simulink model "EKF"  (R2020a)
settings: Solver=VariableStepAuto  StartTime=0.0  StopTime=160  RelTol=1e-3
model workspace (MAT data in the model file):
  Mav0_init = Simulink.Parameter
  Mav0_init.Value = [0.515356; 1.996773; 0.971104; -0.002276; -0.009616; -0.005214; 0.161996; 0.789985; -0.205376; 0.554528; 0; 0; 0; 0; 0; 0; 1; 1; 1; 1; 1; 1; 0; 0; -9.81]
  Mav0_init.DataType = 'auto'
  Mav0_init.Dimensions = [25 1]
  dT = Simulink.Parameter
  dT.Value = 0.01
  dT.DataType = 'auto'
  dT.Dimensions = [1 1]
  g_n = Simulink.Parameter
  g_n.Value = -9.807
  g_n.DataType = 'auto'
  g_n.Dimensions = [1 1]
  sig_a = Simulink.Parameter
  sig_a.Value = 0.4
  sig_a.DataType = 'auto'
  sig_a.Dimensions = [1 1]
  sig_w = Simulink.Parameter
  sig_w.Value = 0.03
  sig_w.DataType = 'auto'
  sig_w.Dimensions = [1 1]
  sigma_l = Simulink.Parameter
  sigma_l.Value = 0.3
  sigma_l.DataType = 'auto'
  sigma_l.Dimensions = [1 1]
  sigma_q = Simulink.Parameter
  sigma_q.Value = 0.05
  sigma_q.DataType = 'auto'
  sigma_q.Dimensions = [1 1]
  sigma_u = Simulink.Parameter
  sigma_u.Value = 0.05
  sigma_u.DataType = 'auto'
  sigma_u.Dimensions = [1 1]
  sigma_u_res = Simulink.Parameter
  sigma_u_res.Value = 0.05
  sigma_u_res.DataType = 'auto'
  sigma_u_res.Dimensions = [1 1]
undefined symbols (not defined in the file or in its folder): Init, no_switchoff
libraries: commchan3 x3
settings Model: OrderedModelArguments=off  Creator=lorenzocollodi  LastModifiedBy=lorenzocollodi

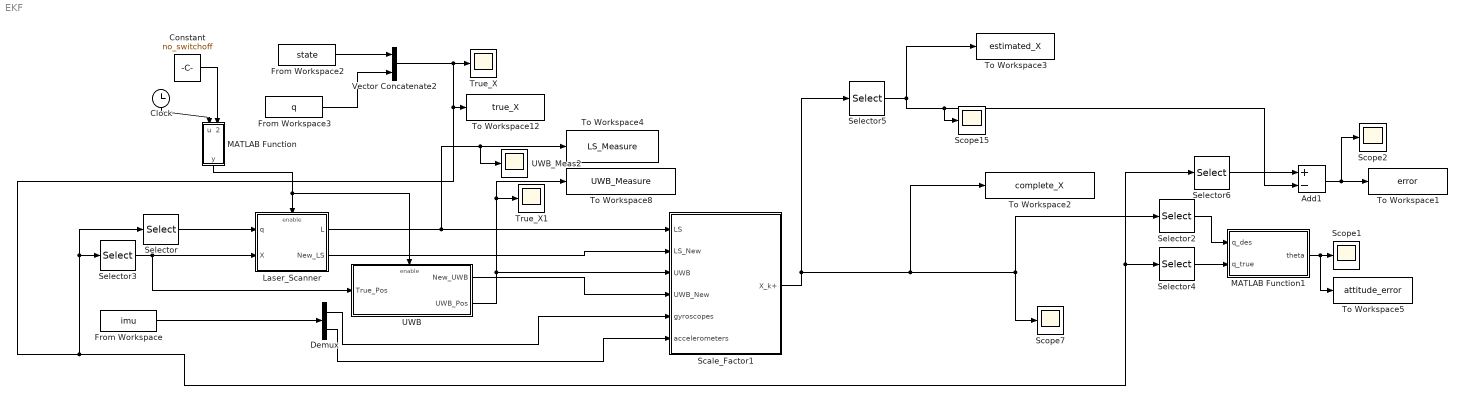
== system EKF ==
  Add1 : Sum  Inputs=+-
  Clock : Clock
  Constant : Constant  Value=no_switchoff
  Demux : Demux  Outputs=2
  From Workspace : FromWorkspace  VariableName=imu
  From Workspace2 : FromWorkspace  VariableName=state
  From Workspace3 : FromWorkspace  VariableName=q  ZeroCross=off
  Laser_Scanner : Subsystem
  MATLAB Function : MATLAB Function  TreatAsAtomicUnit=on
  MATLAB Function1 : MATLAB Function  TreatAsAtomicUnit=on
  Scale_Factor1 : Subsystem
  Scope{1..2,7,15} (4 alike) : Scope
  Selector : Selector  InputPortWidth=10  IndexOptions=Index vector (dialog)  Indices=[7:10]  OutputSizes=1
  Selector2 : Selector  InputPortWidth=25  IndexOptions=Index vector (dialog)  Indices=[7:10]  OutputSizes=1
  Selector3 : Selector  InputPortWidth=10  IndexOptions=Index vector (dialog)  Indices=[1 2 3]  OutputSizes=1
  Selector4 : Selector  InputPortWidth=10  IndexOptions=Index vector (dialog)  Indices=[7:10]  OutputSizes=1
  Selector5 : Selector  InputPortWidth=25  IndexOptions=Index vector (dialog)  Indices=[1:6]  OutputSizes=1
  Selector6 : Selector  InputPortWidth=10  IndexOptions=Index vector (dialog)  Indices=[1:6]  OutputSizes=1
  To Workspace1 : ToWorkspace  VariableName=error  SaveFormat=Timeseries  SampleTime=0.01
  To Workspace12 : ToWorkspace  VariableName=true_X  SaveFormat=Timeseries  SampleTime=0.01
  To Workspace2 : ToWorkspace  VariableName=complete_X  SaveFormat=Timeseries  SampleTime=0.01
  To Workspace3 : ToWorkspace  VariableName=estimated_X  SaveFormat=Timeseries  SampleTime=0.01
  To Workspace4 : ToWorkspace  VariableName=LS_Measure  SaveFormat=Timeseries  SampleTime=0.01
  To Workspace5 : ToWorkspace  VariableName=attitude_error  SaveFormat=Timeseries  SampleTime=0.01
  To Workspace8 : ToWorkspace  VariableName=UWB_Measure  SaveFormat=Timeseries  SampleTime=0.01
  True_X : Scope
  True_X1 : Scope
  UWB : Subsystem
  UWB_Meas2 : Scope
  Vector Concatenate2 : Concatenate
  wires:
  UWB/1(New_UWB) -> Scale_Factor1/4(UWB_New)
  Selector5/1 -> To Workspace3/1, Scope15/1, Add1/2
  Scale_Factor1/1(X_k+) -> To Workspace2/1, Scope7/1, Selector2/1, Selector5/1
  Laser_Scanner/2(New_LS) -> Scale_Factor1/2(LS_New)
  UWB/2(UWB_Pos) -> True_X1/1, To Workspace8/1, Scale_Factor1/3(UWB)
  Add1/1 -> Scope2/1, To Workspace1/1
  From Workspace2/1 -> Vector Concatenate2/1
  Demux/1 -> Scale_Factor1/5(gyroscopes)
  Selector4/1 -> MATLAB Function1/2(q_true)
  Selector6/1 -> Add1/1
  MATLAB Function/1(y) -> UWB/Enable, Laser_Scanner/Enable
  Demux/2 -> Scale_Factor1/6(accelerometers)
  Selector3/1 -> UWB/1(True_Pos), Laser_Scanner/2(X)
  Laser_Scanner/1(L) -> To Workspace4/1, UWB_Meas2/1, Scale_Factor1/1(LS)
  Selector2/1 -> MATLAB Function1/1(q_des)
  Vector Concatenate2/1 -> Selector6/1, Selector4/1, Selector3/1, Selector/1, To Workspace12/1, True_X/1
  MATLAB Function1/1(theta) -> To Workspace5/1, Scope1/1
  From Workspace3/1 -> Vector Concatenate2/2
  From Workspace/1 -> Demux/1
  Clock/1 -> MATLAB Function/1(u)
  Selector/1 -> Laser_Scanner/1(q)
  Constant/1 -> MATLAB Function/2(no_switchoff)

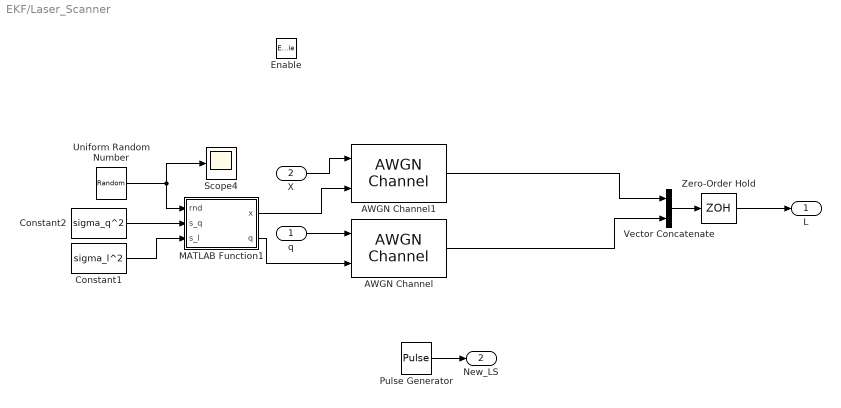
== system EKF/Laser_Scanner ==
  q : Inport  SampleTime=0.005
  X : Inport  Port=2  SampleTime=0.005
  Enable : EnablePort  StatesWhenEnabling=reset
  AWGN Channel : commchan3/AWGN Channel  InputProcessing=Columns as channels (frame based)  seed=53  noiseMode=Variance from port  EbNodB=10  EsNodB=10  SNRdB=10  bitsPerSym=1  Ps=1  Tsym=1  variance=sigma_q^2
  AWGN Channel1 : commchan3/AWGN Channel  InputProcessing=Columns as channels (frame based)  seed=123  noiseMode=Variance from port  EbNodB=10  EsNodB=10  SNRdB=10  bitsPerSym=1  Ps=1  Tsym=1  variance=sigma_l^2
  Constant1 : Constant  Value=sigma_l^2
  Constant2 : Constant  Value=sigma_q^2
  MATLAB Function1 : MATLAB Function  TreatAsAtomicUnit=on
  Pulse Generator : DiscretePulseGenerator  PulseType=Time based  Period=0.1  PulseWidth=5  PhaseDelay=0.1
  Scope4 : Scope
  Uniform Random Number : UniformRandomNumber  Minimum=0  SampleTime=0.1
  Vector Concatenate : Concatenate
  Zero-Order Hold : ZeroOrderHold  SampleTime=0.1
  L : Outport  SampleTime=0.005
  New_LS : Outport  Port=2  SampleTime=0.005  InitialOutput=0
  wires:
  X/1 -> AWGN Channel1/1
  Pulse Generator/1 -> New_LS/1
  Vector Concatenate/1 -> Zero-Order Hold/1
  AWGN Channel1/1 -> Vector Concatenate/1
  Zero-Order Hold/1 -> L/1
  Uniform Random Number/1 -> Scope4/1, MATLAB Function1/1(rnd)
  MATLAB Function1/1(x) -> AWGN Channel1/2
  MATLAB Function1/2(q) -> AWGN Channel/2
  q/1 -> AWGN Channel/1
  AWGN Channel/1 -> Vector Concatenate/2
  Constant2/1 -> MATLAB Function1/2(s_q)
  Constant1/1 -> MATLAB Function1/3(s_l)

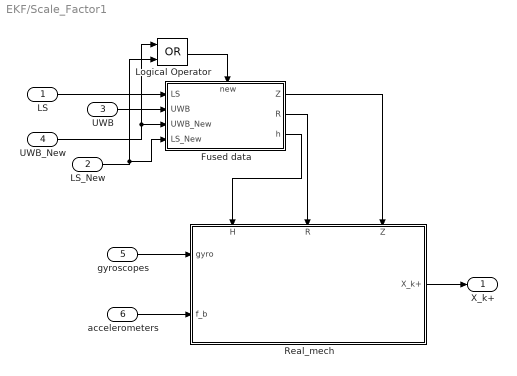
== system EKF/Scale_Factor1 ==
  LS : Inport  SampleTime=0.005
  LS_New : Inport  Port=2  SampleTime=0.005
  UWB : Inport  Port=3  SampleTime=0.005
  UWB_New : Inport  Port=4  SampleTime=0.005
  gyroscopes : Inport  Port=5  SampleTime=0.005
  accelerometers : Inport  Port=6  SampleTime=0.005
  Fused data : Subsystem
      settings: PortSchema="{\"entries\":[{\"content\":{\"sides\":[{\"content\":{\"connectorIds\":[\"In1\",\"In2\",\"In3\",\"In4\"]},\"type\":\"ConnectorPlacement.EquallySpacedRectSide\",\"uuid\":\"3f1f864a-0375-4254-b0e5-a3ccef78d94b\"},{\"content\":{\"connectorIds\":[\"Out1\",\"Out2\",\"Out3\"],\"side\":\"RIGHT\"},\"type\":\"ConnectorPlacement.EquallySpacedRectSide\",\"uuid\":\"a0a53594-1cb6-457a-b6d6-466f13dde723\"},{\"content\":{\"connectorIds\":[\"In5\"],\"side\":\"TOP\"},\"type\":\"ConnectorPlacement.EquallySpacedRectSide\",\"uuid\":\"6845f56e-1f73-40df-9b1b-67b0b5fba5c0\"}]},\"type\":\"ConnectorPlacement.EquallySpacedConnector\",\"uuid\":\"e6a25399-179c-4a75-bf96-00b096d7750c\"}],\"packageUris\":[\"http://schema.mathworks.com/mf0/Connector/19700101\"],\"version\":\"1.0\"}"
  Logical Operator : Logic  Operator=OR  AllPortsSameDT=off  OutDataTypeStr=boolean
  Real_mech : Subsystem
      settings: PortSchema="{\"entries\":[{\"content\":{\"sides\":[{\"content\":{\"connectorIds\":[\"In1\",\"In2\"]},\"type\":\"ConnectorPlacement.EquallySpacedRectSide\",\"uuid\":\"f4a09739-15c6-4b87-9129-8eaded998bc8\"},{\"content\":{\"connectorIds\":[\"Out1\"],\"side\":\"RIGHT\"},\"type\":\"ConnectorPlacement.EquallySpacedRectSide\",\"uuid\":\"b65aee05-6731-4b1e-8841-18a97eaa40b2\"},{\"content\":{\"connectorIds\":[\"In3\",\"In4\",\"In5\"],\"side\":\"TOP\"},\"type\":\"ConnectorPlacement.EquallySpacedRectSide\",\"uuid\":\"6689e3e2-b7bb-4bc5-8dd6-d15d67eac7bb\"}]},\"type\":\"ConnectorPlacement.EquallySpacedConnector\",\"uuid\":\"d04e917e-36a5-4a97-9f44-5590d0d9db30\"}],\"packageUris\":[\"http://schema.mathworks.com/mf0/Connector/19700101\"],\"version\":\"1.0\"}"
  X_k+ : Outport  SampleTime=0.005
  wires:
  UWB/1 -> Fused data/2(UWB)
  accelerometers/1 -> Real_mech/2(f_b)
  Real_mech/1(X_k+) -> X_k+/1
  gyroscopes/1 -> Real_mech/1(gyro)
  LS_New/1 -> Fused data/4(LS_New), Logical Operator/2
  UWB_New/1 -> Logical Operator/1, Fused data/3(UWB_New)
  Fused data/1(Z) -> Real_mech/5(Z)
  Fused data/2(R) -> Real_mech/4(R)
  Fused data/3(h) -> Real_mech/3(H)
  LS/1 -> Fused data/1(LS)
  Logical Operator/1 -> Fused data/5(new)

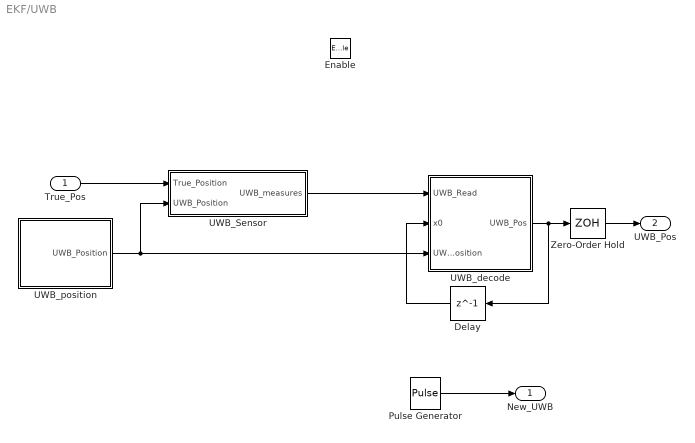
== system EKF/UWB ==
  True_Pos : Inport  SampleTime=0.005
  Enable : EnablePort
  Delay : Delay  DelayLength=1  InitialCondition=[0; 0; 0]  SampleTime=0.1
  Pulse Generator : DiscretePulseGenerator  PulseType=Time based  Period=0.1  PulseWidth=5  PhaseDelay=0.1
  UWB_Sensor : Subsystem
  UWB_decode : Subsystem
  UWB_position : Subsystem
  Zero-Order Hold : ZeroOrderHold  SampleTime=0.1
  New_UWB : Outport  SampleTime=0.005  InitialOutput=0
  UWB_Pos : Outport  Port=2  SampleTime=0.005
  wires:
  True_Pos/1 -> UWB_Sensor/1(True_Position)
  UWB_Sensor/1(UWB_measures) -> UWB_decode/1(UWB_Read)
  UWB_position/1(UWB_Position) -> UWB_Sensor/2(UWB_Position), UWB_decode/3(UWB_Position)
  Delay/1 -> UWB_decode/2(x0)
  UWB_decode/1(UWB_Pos) -> Zero-Order Hold/1, Delay/1
  Pulse Generator/1 -> New_UWB/1
  Zero-Order Hold/1 -> UWB_Pos/1

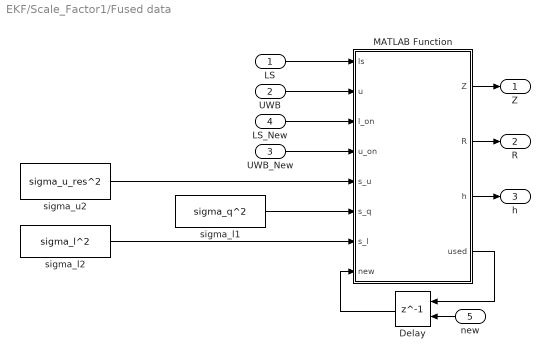
== system EKF/Scale_Factor1/Fused data ==
  LS : Inport  SampleTime=0.005
  UWB : Inport  Port=2  SampleTime=0.005
  UWB_New : Inport  Port=3  SampleTime=0.005
  LS_New : Inport  Port=4  SampleTime=0.005
  new : Inport  Port=5  SampleTime=0.005
  Delay : Delay  DelayLength=1  InitialCondition=1  ExternalReset=Rising  SampleTime=0.005
      settings: InputPortMap=u0,r5
  MATLAB Function : MATLAB Function  TreatAsAtomicUnit=on
  sigma_l1 : Constant  Value=sigma_q^2
  sigma_l2 : Constant  Value=sigma_l^2
  sigma_u2 : Constant  Value=sigma_u_res^2
  Z : Outport  SampleTime=0.005
  R : Outport  Port=2  SampleTime=0.005
  h : Outport  Port=3  SampleTime=0.005
  wires:
  LS/1 -> MATLAB Function/1(ls)
  UWB/1 -> MATLAB Function/2(u)
  UWB_New/1 -> MATLAB Function/4(u_on)
  sigma_u2/1 -> MATLAB Function/5(s_u)
  sigma_l2/1 -> MATLAB Function/7(s_l)
  MATLAB Function/1(Z) -> Z/1
  MATLAB Function/2(R) -> R/1
  MATLAB Function/3(h) -> h/1
  MATLAB Function/4(used) -> Delay/1
  Delay/1 -> MATLAB Function/8(new)
  new/1 -> Delay/2
  sigma_l1/1 -> MATLAB Function/6(s_q)
  LS_New/1 -> MATLAB Function/3(l_on)

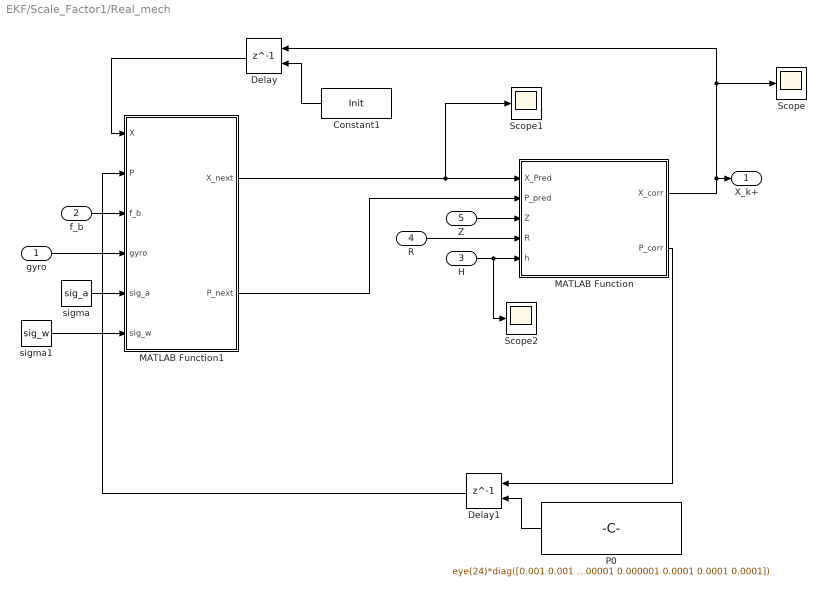
== system EKF/Scale_Factor1/Real_mech ==
  gyro : Inport  SampleTime=0.005
  f_b : Inport  Port=2  SampleTime=0.005
  H : Inport  Port=3  PortDimensions=[7, 25]  SampleTime=0.005
  R : Inport  Port=4  PortDimensions=[7,7]  SampleTime=0.005
  Z : Inport  Port=5  SampleTime=0.005
  Constant1 : Constant  Value=Init
  Delay : Delay  DelayLength=1  InitialConditionSource=Input port  InitialCondition=[0.515356;1.996773;0.971104;-0.002276;-0.009616;-0.005214; 0; 0; -9.81]  SampleTime=0.005
      settings: InputPortMap=u0,p4
  Delay1 : Delay  DelayLength=1  InitialConditionSource=Input port  InitialCondition=0  SampleTime=0.005
      settings: InputPortMap=u0,p4
  MATLAB Function : MATLAB Function  TreatAsAtomicUnit=on
  MATLAB Function1 : MATLAB Function  TreatAsAtomicUnit=on
  P0 : Constant  Value=eye(24)*diag([0.001 0.001 0.001 0.001 0.001 0.001 0.0001 0.0001 0.0001 0.0001 0.001 0.001 0.001 0.000001 0.000001 0.0000001 0.000001 0.000001 0.000001 0.000001 0.000001 0.0001 0.0001 0.0001])
  Scope : Scope
  Scope1 : Scope
  Scope2 : Scope
  sigma : Constant  Value=sig_a  SampleTime=0.01
  sigma1 : Constant  Value=sig_w  SampleTime=0.01
  X_k+ : Outport  SampleTime=0.005
  wires:
  sigma1/1 -> MATLAB Function1/6(sig_w)
  MATLAB Function/1(X_corr) -> Delay/1, Scope/1, X_k+/1
  Delay/1 -> MATLAB Function1/1(X)
  Delay1/1 -> MATLAB Function1/2(P)
  gyro/1 -> MATLAB Function1/4(gyro)
  P0/1 -> Delay1/2
  R/1 -> MATLAB Function/4(R)
  Z/1 -> MATLAB Function/3(Z)
  H/1 -> Scope2/1, MATLAB Function/5(h)
  Constant1/1 -> Delay/2
  f_b/1 -> MATLAB Function1/3(f_b)
  MATLAB Function1/2(P_next) -> MATLAB Function/2(P_pred)
  sigma/1 -> MATLAB Function1/5(sig_a)
  MATLAB Function1/1(X_next) -> Scope1/1, MATLAB Function/1(X_Pred)
  MATLAB Function/2(P_corr) -> Delay1/1

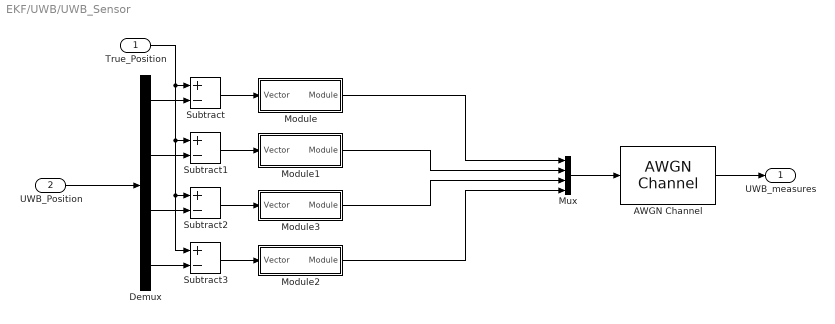
== system EKF/UWB/UWB_Sensor ==
  True_Position : Inport
  UWB_Position : Inport  Port=2
  AWGN Channel : commchan3/AWGN Channel  InputProcessing=Columns as channels (frame based)  seed=13561  noiseMode=Variance from mask  EbNodB=10  EsNodB=10  SNRdB=10  bitsPerSym=1  Ps=1  Tsym=1  variance=sigma_u^2
  Demux : Demux
  Module : Subsystem
  Module1 : Subsystem
  Module2 : Subsystem
  Module3 : Subsystem
  Mux : Mux
  Subtract{,1..3} (4 alike) : Sum  Inputs=+-
  UWB_measures : Outport  PortDimensions=4
  wires:
  UWB_Position/1 -> Demux/1
  Demux/1 -> Subtract/2
  Demux/4 -> Subtract3/2
  Demux/3 -> Subtract2/2
  Demux/2 -> Subtract1/2
  True_Position/1 -> Subtract2/1, Subtract3/1, Subtract1/1, Subtract/1
  Subtract/1 -> Module/1(Vector)
  Subtract3/1 -> Module2/1(Vector)
  Subtract2/1 -> Module3/1(Vector)
  Subtract1/1 -> Module1/1(Vector)
  Mux/1 -> AWGN Channel/1
  AWGN Channel/1 -> UWB_measures/1
  Module/1(Module) -> Mux/1
  Module1/1(Module) -> Mux/2
  Module3/1(Module) -> Mux/3
  Module2/1(Module) -> Mux/4

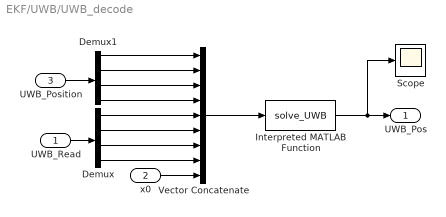
== system EKF/UWB/UWB_decode ==
  UWB_Read : Inport  PortDimensions=4  SampleTime=10*dT
  x0 : Inport  Port=2  PortDimensions=3  SampleTime=10*dT
  UWB_Position : Inport  Port=3  SampleTime=10*dT
  Demux : Demux
  Demux1 : Demux
  Interpreted MATLAB Function : MATLABFcn  MATLABFcn=solve_UWB  OutputDimensions=3
  Scope : Scope
  Vector Concatenate : Concatenate  NumInputs=9
  UWB_Pos : Outport  PortDimensions=3  SampleTime=0.1
  wires:
  UWB_Read/1 -> Demux/1
  Demux1/1 -> Vector Concatenate/1
  Demux1/2 -> Vector Concatenate/2
  Demux1/3 -> Vector Concatenate/3
  Demux1/4 -> Vector Concatenate/4
  Demux/1 -> Vector Concatenate/5
  Demux/2 -> Vector Concatenate/6
  Demux/3 -> Vector Concatenate/7
  Demux/4 -> Vector Concatenate/8
  Interpreted MATLAB Function/1 -> Scope/1, UWB_Pos/1
  x0/1 -> Vector Concatenate/9
  UWB_Position/1 -> Demux1/1
  Vector Concatenate/1 -> Interpreted MATLAB Function/1

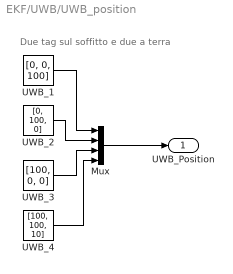
== system EKF/UWB/UWB_position ==
  note: Due tag sul soffitto e due a terra
  Mux : Mux
  UWB_1 : Constant  Value=[0, 0, 100]
  UWB_2 : Constant  Value=[0, 100, 0]
  UWB_3 : Constant  Value=[100, 0, 0]
  UWB_4 : Constant  Value=[100, 100, 10]
  UWB_Position : Outport
  wires:
  UWB_3/1 -> Mux/3
  Mux/1 -> UWB_Position/1
  UWB_4/1 -> Mux/4
  UWB_1/1 -> Mux/1
  UWB_2/1 -> Mux/2

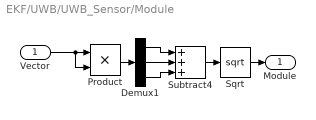
== system EKF/UWB/UWB_Sensor/Module ==
  Vector : Inport
  Demux1 : Demux  Outputs=3
  Product : Product
  Sqrt : Sqrt  SaturateOnIntegerOverflow=on
  Subtract4 : Sum  Inputs=+++
  Module : Outport  PortDimensions=1
  wires:
  Subtract4/1 -> Sqrt/1
  Vector/1 -> Product/2, Product/1
  Product/1 -> Demux1/1
  Demux1/1 -> Subtract4/1
  Demux1/3 -> Subtract4/3
  Demux1/2 -> Subtract4/2
  Sqrt/1 -> Module/1

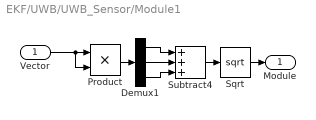
== system EKF/UWB/UWB_Sensor/Module1 ==
  Vector : Inport
  Demux1 : Demux  Outputs=3
  Product : Product
  Sqrt : Sqrt  SaturateOnIntegerOverflow=on
  Subtract4 : Sum  Inputs=+++
  Module : Outport  PortDimensions=1
  wires:
  Demux1/3 -> Subtract4/3
  Subtract4/1 -> Sqrt/1
  Product/1 -> Demux1/1
  Sqrt/1 -> Module/1
  Demux1/1 -> Subtract4/1
  Vector/1 -> Product/2, Product/1
  Demux1/2 -> Subtract4/2

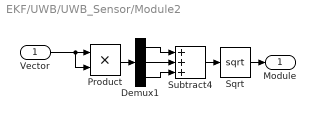
== system EKF/UWB/UWB_Sensor/Module2 ==
  Vector : Inport
  Demux1 : Demux  Outputs=3
  Product : Product
  Sqrt : Sqrt  SaturateOnIntegerOverflow=on
  Subtract4 : Sum  Inputs=+++
  Module : Outport  PortDimensions=1
  wires:
  Demux1/3 -> Subtract4/3
  Subtract4/1 -> Sqrt/1
  Product/1 -> Demux1/1
  Sqrt/1 -> Module/1
  Demux1/1 -> Subtract4/1
  Vector/1 -> Product/2, Product/1
  Demux1/2 -> Subtract4/2

== system EKF/UWB/UWB_Sensor/Module3 ==
  Vector : Inport
  Demux1 : Demux  Outputs=3
  Product : Product
  Sqrt : Sqrt  SaturateOnIntegerOverflow=on
  Subtract4 : Sum  Inputs=+++
  Module : Outport  PortDimensions=1
  wires:
  Demux1/3 -> Subtract4/3
  Subtract4/1 -> Sqrt/1
  Product/1 -> Demux1/1
  Sqrt/1 -> Module/1
  Demux1/1 -> Subtract4/1
  Vector/1 -> Product/2, Product/1
  Demux1/2 -> Subtract4/2

== matlab function EKF/MATLAB Function ==
  data: u input; y output; no_switchoff input
function y = fcn(u, no_switchoff)
if u < 50
    y = 1;
elseif u<60
    y = 0;
else
    y = 1;
end
if no_switchoff
    y = 1;
end
end

== matlab function EKF/MATLAB Function1 ==
  data: q_des input; theta output; q_true input
function theta  = derivative(q_des, q_true)
%transform_BN: takes as input the orientation of the UAV as RPY (from
% mechanization). Returns the matrix that transforms from body frame
% to navigation frame

a = q_des(1);
b = q_des(2);
c = q_des(3);
d = q_des(4);

m_11 = a;
m_12 = -b;
m_13 = -c;
m_14 = -d;
m_21 = b;
m_22 = a;
m_23 = -d;
m_24 = c;
m_31 = c;
m_32 = d;
m_33 = a;
m_34 = -b;
m_41 = d;
m_42 = -c;
m_43 = b;
m_44 = a;

matrix = [[m_11 m_12 m_13 m_14]; [m_21 m_22 m_23 m_24]; [m_31 m_32 m_33 m_34]; [m_41 m_42 m_43 m_44]];
diff = matrix*[q_true(1); -q_true(2:4)];
theta = 2*atan2(norm(diff(2:4)), diff(1));
if theta > pi
    theta = 2*pi - theta;
end
end

== matlab function EKF/Laser_Scanner/MATLAB Function1 ==
  data: x output; rnd input; q output; s_q input; s_l input
function [x, q]= fcn(rnd, s_q, s_l)
if rnd > 0.995
    q = s_q*5;
    x = 9*s_l*5;
else
    q = s_q;
    x = 9*s_l;
end
end

== matlab function EKF/Scale_Factor1/Fused data/MATLAB Function ==
  data: ls input; u input; Z output; l_on input; u_on input; s_u input; s_q input; s_l input; R output; h output; used output; new input
function [Z, R, h, used]= fcn(ls, u, l_on, u_on, s_u, s_q, s_l,new)
l = ls(1:3);
q = ls(4:7);
if l_on && u_on
    x = (l*s_u + u*s_l)/(s_u+s_l);
    Z = [x; q];
    h = [eye(3) zeros([3 22]); zeros([4 6]) eye(4) zeros([4 15])];
    s_mean = (s_u*s_l)/(s_u+s_l);
    R = eye(7)*diag([s_mean; s_mean; s_mean; s_q; s_q; s_q; s_q]);
elseif l_on
    Z = [l; q];
    h = [eye(3) zeros([3 22]); zeros([4 6]) eye(4) zeros([4 15])];
    R = eye(7)*diag([s_l; s_l; s_l; s_q; s_q; s_q; s_q]);
elseif u_on
    Z = [u; q];
    h = [eye(3) zeros([3 22]); zeros([4 25])];
    R = eye(7)*diag([s_u; s_u; s_u; s_q; s_q; s_q; s_q]);
else
    Z = [u; q];
    R = eye(7);
    h = zeros([7 25]);
end
if new == 0
    Z = [u; q];
    R = eye(7);
    h = zeros([7 25]);
end
used = 0;
end

== matlab function EKF/Scale_Factor1/Real_mech/MATLAB Function ==
  data: X_corr output; X_Pred input; P_pred input; P_corr output; Z input; R input; h input
function [X_corr, P_corr] = correction(X_Pred, P_pred, Z, R, h)
I = eye(24);
q = X_Pred(7:10);
X_corr = X_Pred;
a = q(1);
b = q(2);
c = q(3);
d = q(4);

m_12 = -b;
m_13 = -c;
m_14 = -d;
m_22 = a;
m_23 = -d;
m_24 = c;
m_32 = d;
m_33 = a;
m_34 = -b;
m_42 = -c;
m_43 = b;
m_44 = a;

matrix = [[m_12 m_13 m_14]; [m_22 m_23 m_24]; [m_32 m_33 m_34]; [m_42 m_43 m_44]]/2;

if h(1, 1) ~= 0
    h(1, 1) = h(1, 1);
end
Hx = zeros([25 24]);
Hx(1:6, 1:6) = eye(6);
Hx(7:10, 7:9) = matrix; 
Hx(11:25, 10:24) = eye(15);
H = h*Hx;
K = P_pred*(H.')/(H*P_pred*(H.')+R);
Z(4:7) = Z(4:7)/norm(Z(4:7));
Res = (Z - h*X_Pred);
%q_f = Z(4:7);
%q_f = q_f/norm(q_f);
%q_i_c = [q(1); -q(2:4)];
%q_v = [q_f(1) -q_f(2) -q_f(3) -q_f(4); q_f(2) q_f(1) -q_f(4) q_f(3);q_f(3) q_f(4) q_f(1) -q_f(2);q_f(4) -q_f(3) q_f(2) q_f(1)];
%Res(4:7) = q_v*q_i_c;
dX = K*Res;
P_corr = (I - K*H)*P_pred;
X_corr(1:6) = X_Pred(1:6) + dX(1:6);
X_corr(11:25) = X_Pred(11:25) + dX(10:24);
w = dX(7:9);
if w == [0; 0; 0]
    dq = [1; 0; 0; 0];
else
    theta = norm(w);
    v = w/norm(w);
    dq = [cos(theta/2); v*sin(theta/2)];
end
q_vett = [q(1) -q(2) -q(3) -q(4); q(2) q(1) -q(4) q(3);q(3) q(4) q(1) -q(2);q(4) -q(3) q(2) q(1)];
G = eye(24);
dG = cross(repmat(w/2,1,3),eye(3,3));
G(7:9, 7:9) = G(7:9, 7:9) - dG;
P_corr = G*P_corr*G.';
X_corr(7:10) = q_vett*dq;
end

== matlab function EKF/Scale_Factor1/Real_mech/MATLAB Function1 ==
  data: X input; P input; f_b input; gyro input; X_next output; P_next output; sig_a input; sig_w input
function [X_next, P_next] = predict(X, P, f_b, gyro, sig_a, sig_w)
%transform_BN: takes as input the orientation of the UAV as RPY (from
% mechanization). Returns the matrix that transforms from body frame
% to navigation frame
X_next = X;

q = X(7:10);
p = X(1:3);
v = X(4:6);
ba = X(11:13);
bw = X(14:16);
Sa = diag(X(17:19));
Sw = diag(X(20:22));
g = X(23:25);

a = q(1);
b = q(2);
c = q(3);
d = q(4);

m_11 = a^2+b^2-c^2-d^2;
m_12 = 2*(b*c-a*d);
m_13 = 2*(b*d+a*c);
m_21 = 2*(b*c+a*d);
m_22 = a^2-b^2+c^2-d^2;
m_23 = 2*(c*d-a*b);
m_31 = 2*(b*d-a*c);
m_32 = 2*(c*d+a*b);
m_33 = a^2-b^2-c^2+d^2;

C_bn = [[m_11 m_12 m_13]; [m_21 m_22 m_23]; [m_31 m_32 m_33]];
X_next(1:3) = p + v*0.005 + ((C_bn/Sa)*(f_b-ba)+g)*0.005*0.005/2;
X_next(4:6) = v + ((C_bn/Sa)*(f_b-ba) + g)*0.005;
w = Sw\(gyro - bw);
theta = norm(w)*0.005;
v = w/norm(w);
dq = [cos(theta/2); v*sin(theta/2)];
q_vett = [q(1) -q(2) -q(3) -q(4); q(2) q(1) -q(4) q(3);q(3) q(4) q(1) -q(2); q(4) -q(3) q(2) q(1)];
X_next(7:10) = q_vett*dq;
Q = diag([sig_a^2*0.005^2 sig_a^2*0.005^2 sig_a^2*0.005^2 sig_w^2*0.005^2 sig_w^2*0.005^2 sig_w^2*0.005^2 0.00001*0.005 0.00001*0.005 0.00001*0.005 0.00001*0.005 0.00001*0.005 0.00001*0.005]);
Fi = [zeros([3 3]) eye(3)*(0.005^2)/2 zeros([3 6]); eye(12); zeros([9 12])];

a = dq(1);
b = dq(2);
c = dq(3);
d = dq(4);

m_11 = a^2+b^2-c^2-d^2;
m_12 = 2*(b*c-a*d);
m_13 = 2*(b*d+a*c);
m_21 = 2*(b*c+a*d);
m_22 = a^2-b^2+c^2-d^2;
m_23 = 2*(c*d-a*b);
m_31 = 2*(b*d-a*c);
m_32 = 2*(c*d+a*b);
m_33 = a^2-b^2-c^2+d^2;

R = [[m_11 m_12 m_13]; [m_21 m_22 m_23]; [m_31 m_32 m_33]];


Fx = eye(24);
a_true = Sa\(f_b-ba);
a_vett = cross(repmat(a_true,1,3),eye(3,3));
Fx(1:3, 4:6) = eye(3)*0.005;
Fx(4:6, 7:9) = -C_bn*a_vett*0.005;
Fx(4:6, 10:12) = -(C_bn/Sa)*0.005;
Fx(4:6, 16:18) = -diag(a_true)/Sa*0.005;
Fx(4:6, 22:24) = eye(3)*0.005;
Fx(1:3, 7:12) = Fx(4:6, 7:12)*0.005/2;
Fx(1:3, 16:18) = Fx(4:6, 16:18)*0.005/2;
Fx(1:3, 22:24) = Fx(4:6, 22:24)*0.005/2;
Fx(7:9, 7:9) = R.';
Fx(7:9, 13:15) = -Sw\eye(3)*0.005;
Fx(7:9, 19:21) = -Sw\diag(w)*0.005;

P_next = Fx*P*Fx.' + Fi*Q*Fi.';
end
